simulink model "WT_FFNN_trainbfg_15_15_15_st_5_controller_Oct_6_2023_Nor_0"  (R2021a)
settings: Solver=VariableStepAuto  StartTime=0.0  StopTime=10.0  RelTol=1e-3
libraries: neural x50
(part 2 of 2)

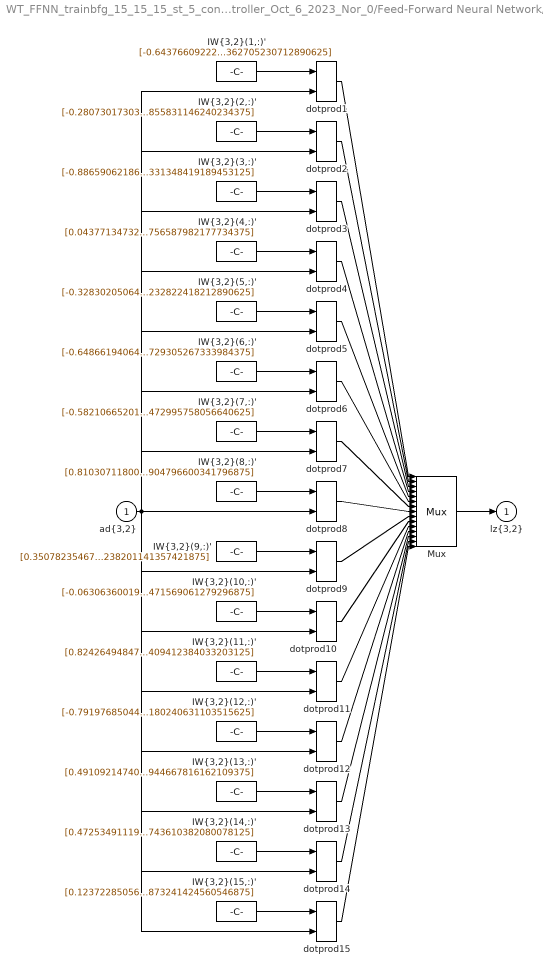
== system WT_FFNN_trainbfg_15_15_15_st_5_controller_Oct_6_2023_Nor_0/Feed-Forward Neural Network/Layer 3/LW{3,2} ==
  "ad{3,2}" : Inport  PortDimensions=15
      mask Display: e = 0.06;c1 = [120 230 180]/255;c2 = ([120 230 180]+0)/(256+128);c3 = ([120 230 180]+128)/(256+128);patch([0 1 1 0],[0 0 1 1],c1);patch([0 1 1 1-e 1-e 0+e],[0 0 1 1-e 0+e 0+e],c2);patch([0 0 1 1-e 0+e 0+e],[0 1 1 1-e 1-e 0+e],c3);plot([0 1 1 0 0],[0 0 1 1 0]);
  "IW{3,2}(1,:)'" : Constant  Value=[-0.643766092226467190329231016221456229686737060546875;-0.63161180496894697711240951321087777614593505859375;-0.0878846663125170124430951545946300029754638671875;0.0675439035340004156893201070488430559635162353515625;0.3850639727730376105085952076478861272335052490234375;-0.897336227775257899708094555535353720188140869140625;0.4800646559755552544856982422061264514923095703125;-0.5886509570704803184781894742627628147602081298828125;-0.7754320756879466980393544872640632092952728271484375;-0.0247924491321527273868241536547429859638214111328125;-0.81529532256159686909313677460886538028717041015625;-0.367142001707418064171406513196416199207305908203125;0.9758694699049907939070180873386561870574951171875;-0.2984465102282147785928145822254009544849395751953125;-0.750254482560374302835271009826101362705230712890625]
      mask Display: e = 0.06;c1 = [120 150 230]/255;c2 = ([120 150 230]+0)/383;c3 = ([120 150 230]+128)/383;patch([0 1 1 0],[0 0 1 1],c1);patch([0 1 1 1-e 1-e 0+e],[0 0 1 1-e 0+e 0+e],c2);patch([0 0 1 1-e 0+e 0+e],[0 1 1 1-e 1-e 0+e],c3);plot([0 1 1 0 0],[0 0 1 1 0]);disp('weights');
  "IW{3,2}(10,:)'" : Constant  Value=[-0.0630636001920052979841102569480426609516143798828125;-0.366578988970010344328187557039200328290462493896484375;0.519459618514004350942059318185783922672271728515625;0.0921458484020575563366861615577363409101963043212890625;-0.7442232404340096696415685073588974773883819580078125;-1.079327489691291219742197426967322826385498046875;0.369217770489993657445637609271216206252574920654296875;-0.601335359818960579758595486055128276348114013671875;0.0032313445087976890197911661317675680038519203662872314453125;-0.896971085063572370899009911227039992809295654296875;-0.6861878613530782988760847729281522333621978759765625;0.68989207606787716908769425572245381772518157958984375;0.07321916960369133364761040638768463395535945892333984375;-0.333963203642246353464173580505303107202053070068359375;0.52767289553089458120638255422818474471569061279296875]
      mask Display: e = 0.06;c1 = [120 150 230]/255;c2 = ([120 150 230]+0)/383;c3 = ([120 150 230]+128)/383;patch([0 1 1 0],[0 0 1 1],c1);patch([0 1 1 1-e 1-e 0+e],[0 0 1 1-e 0+e 0+e],c2);patch([0 0 1 1-e 0+e 0+e],[0 1 1 1-e 1-e 0+e],c3);plot([0 1 1 0 0],[0 0 1 1 0]);disp('weights');
  "IW{3,2}(11,:)'" : Constant  Value=[0.82426494847924569597807931131683290004730224609375;-0.97294544089362500205453443413716740906238555908203125;0.28985203172992990428014081771834753453731536865234375;0.0548147619280814624165287796131451614201068878173828125;0.0990802140303959077982653980143368244171142578125;0.292797576551611538064889828092418611049652099609375;0.58356272391747465722033894053311087191104888916015625;-0.5219904965795241214010502517339773476123809814453125;-0.7694257985340786643035926317679695785045623779296875;-0.3683771233222679075680616733734495937824249267578125;-0.79654204929376859478651340396027080714702606201171875;0.437512109004076332752219968824647367000579833984375;-0.69209100898033104609652355065918527543544769287109375;-0.2746468641281059053227409094688482582569122314453125;0.51865325037653786655056364907068200409412384033203125]
      mask Display: e = 0.06;c1 = [120 150 230]/255;c2 = ([120 150 230]+0)/383;c3 = ([120 150 230]+128)/383;patch([0 1 1 0],[0 0 1 1],c1);patch([0 1 1 1-e 1-e 0+e],[0 0 1 1-e 0+e 0+e],c2);patch([0 0 1 1-e 0+e 0+e],[0 1 1 1-e 1-e 0+e],c3);plot([0 1 1 0 0],[0 0 1 1 0]);disp('weights');
  "IW{3,2}(12,:)'" : Constant  Value=[-0.7919768504412429965810815701843239367008209228515625;1.021337337366363673396563171991147100925445556640625;-1.10070096439400533228081258130259811878204345703125;0.54194625703035803621077093339408747851848602294921875;-0.029541182830081336163630112423561513423919677734375;-0.09421701438622749613660545264792745001614093780517578125;-0.57891826972255999717020813477574847638607025146484375;0.08794848163775025040589383706901571713387966156005859375;1.2460687532080745310025804428732953965663909912109375;0.448536259228720146641222754624322988092899322509765625;-0.88810303508568055885774583657621406018733978271484375;-0.1498027423311489580992628134481492452323436737060546875;0.160199994159698155815618747510598041117191314697265625;-0.257260398151900548935344659184920601546764373779296875;0.48137873566461009122718905928195454180240631103515625]
      mask Display: e = 0.06;c1 = [120 150 230]/255;c2 = ([120 150 230]+0)/383;c3 = ([120 150 230]+128)/383;patch([0 1 1 0],[0 0 1 1],c1);patch([0 1 1 1-e 1-e 0+e],[0 0 1 1-e 0+e 0+e],c2);patch([0 0 1 1-e 0+e 0+e],[0 1 1 1-e 1-e 0+e],c3);plot([0 1 1 0 0],[0 0 1 1 0]);disp('weights');
  "IW{3,2}(13,:)'" : Constant  Value=[0.4910921474034346534409678497468121349811553955078125;-0.48744557436756996704474431680864654481410980224609375;-1.014034144660356684397584103862755000591278076171875;0.4724792507893542659047625420498661696910858154296875;0.7809513583688765248069785229745320975780487060546875;0.5203015162644302193939438438974320888519287109375;-0.6241583092029754364915561382076703011989593505859375;-0.81700253732117555927061403053812682628631591796875;-0.6241863057843290985005069160251878201961517333984375;0.2760602048501932248569801231496967375278472900390625;-0.7697405297430404136349579857778735458850860595703125;-0.45085593242650479073319047529366798698902130126953125;-0.439984497093076132312461368201184086501598358154296875;0.554792900069340788604677072726190090179443359375;0.4873766829746519757549094720161519944667816162109375]
      mask Display: e = 0.06;c1 = [120 150 230]/255;c2 = ([120 150 230]+0)/383;c3 = ([120 150 230]+128)/383;patch([0 1 1 0],[0 0 1 1],c1);patch([0 1 1 1-e 1-e 0+e],[0 0 1 1-e 0+e 0+e],c2);patch([0 0 1 1-e 0+e 0+e],[0 1 1 1-e 1-e 0+e],c3);plot([0 1 1 0 0],[0 0 1 1 0]);disp('weights');
  "IW{3,2}(14,:)'" : Constant  Value=[0.4725349111932770629351807656348682940006256103515625;-0.689178476180853039068097132258117198944091796875;0.2356972366457289747021519588088267482817173004150390625;0.626963724406184308435285856830887496471405029296875;0.597920557625758686270955877262167632579803466796875;0.625541261646222590542265606927685439586639404296875;-1.1026078992220214036734660112415440380573272705078125;-0.19770856332119357556820204990799538791179656982421875;-0.077371211188020871940551614898140542209148406982421875;-0.7870523574073573502829503922839649021625518798828125;-0.669477187150147035055169908446259796619415283203125;-0.9783172116776768234558403491973876953125;0.905331492010126748226639392669312655925750732421875;-0.5450102600935970986739675936405546963214874267578125;-0.7881591665344693797834452198003418743610382080078125]
      mask Display: e = 0.06;c1 = [120 150 230]/255;c2 = ([120 150 230]+0)/383;c3 = ([120 150 230]+128)/383;patch([0 1 1 0],[0 0 1 1],c1);patch([0 1 1 1-e 1-e 0+e],[0 0 1 1-e 0+e 0+e],c2);patch([0 0 1 1-e 0+e 0+e],[0 1 1 1-e 1-e 0+e],c3);plot([0 1 1 0 0],[0 0 1 1 0]);disp('weights');
  "IW{3,2}(15,:)'" : Constant  Value=[0.12372285056327481100879595032893121242523193359375;-0.72140085239758067192639146014698781073093414306640625;0.86439986632040366476559256625478155910968780517578125;-0.59112412850498685656930319964885711669921875;0.4686821673919394637408686321577988564968109130859375;-0.258477290842136608883805592995486222207546234130859375;0.7900688209342423551362344369408674538135528564453125;-1.0831855079199177449567059738910757005214691162109375;0.1882682004181205071002835893523297272622585296630859375;-0.761400721393763912914209868176840245723724365234375;-0.29988241519058600470515330016496591269969940185546875;0.11863292152367811704838373998427414335310459136962890625;0.50817119992942860751128364427131600677967071533203125;-0.366864516161464815358073110473924316465854644775390625;0.362897935872615373664729077063384465873241424560546875]
      mask Display: e = 0.06;c1 = [120 150 230]/255;c2 = ([120 150 230]+0)/383;c3 = ([120 150 230]+128)/383;patch([0 1 1 0],[0 0 1 1],c1);patch([0 1 1 1-e 1-e 0+e],[0 0 1 1-e 0+e 0+e],c2);patch([0 0 1 1-e 0+e 0+e],[0 1 1 1-e 1-e 0+e],c3);plot([0 1 1 0 0],[0 0 1 1 0]);disp('weights');
  "IW{3,2}(2,:)'" : Constant  Value=[-0.2807301730358393587749787911889143288135528564453125;0.19442270067570976976867314078845083713531494140625;-0.7966612127504897333807321047061122953891754150390625;-0.7816915759150828701962154809734784066677093505859375;0.1133396699280251329611246546846814453601837158203125;-0.854229401802047760838831891305744647979736328125;-0.530346170504191416483763532596640288829803466796875;-0.2234567379043965740237354111741296947002410888671875;0.5688557814878254514923128226655535399913787841796875;0.5379165281177382684774102017399854958057403564453125;-0.9843594128613302185470956828794442117214202880859375;-0.564873381154358700229067835607565939426422119140625;-0.6591359538862333611319854753674007952213287353515625;0.3710714174950744403957969552720896899700164794921875;-0.951131967899252028786349910660646855831146240234375]
      mask Display: e = 0.06;c1 = [120 150 230]/255;c2 = ([120 150 230]+0)/383;c3 = ([120 150 230]+128)/383;patch([0 1 1 0],[0 0 1 1],c1);patch([0 1 1 1-e 1-e 0+e],[0 0 1 1-e 0+e 0+e],c2);patch([0 0 1 1-e 0+e 0+e],[0 1 1 1-e 1-e 0+e],c3);plot([0 1 1 0 0],[0 0 1 1 0]);disp('weights');
  "IW{3,2}(3,:)'" : Constant  Value=[-0.8865906218634176383375233854167163372039794921875;-0.4173596361538345345110201378702186048030853271484375;0.94817629014061421965919862486771307885646820068359375;0.382433549701703678902475758150103501975536346435546875;-0.20695841483681487460444259340874850749969482421875;-0.9808227906319275657409662017016671597957611083984375;0.472630354818219744483798194778501056134700775146484375;0.1552047080825973146556151505137677304446697235107421875;-0.5535059857181021669703113730065524578094482421875;-0.26582664726738924887428083820850588381290435791015625;-0.1114708427107084232066114282133639790117740631103515625;-0.5343712969343707985814262428903020918369293212890625;-0.55095411778595515528422765783034265041351318359375;-0.421040236130094502886578311517951078712940216064453125;-0.419775850566837693822463961623725481331348419189453125]
      mask Display: e = 0.06;c1 = [120 150 230]/255;c2 = ([120 150 230]+0)/383;c3 = ([120 150 230]+128)/383;patch([0 1 1 0],[0 0 1 1],c1);patch([0 1 1 1-e 1-e 0+e],[0 0 1 1-e 0+e 0+e],c2);patch([0 0 1 1-e 0+e 0+e],[0 1 1 1-e 1-e 0+e],c3);plot([0 1 1 0 0],[0 0 1 1 0]);disp('weights');
  "IW{3,2}(4,:)'" : Constant  Value=[0.0437713473225584959180878286133520305156707763671875;-0.7804216873352183281298266592784784734249114990234375;-0.2787118030579514016409348187153227627277374267578125;-0.201163548237447697974999982761801220476627349853515625;-0.8768186658920706921804821831756271421909332275390625;0.69390680565058027173819255040143616497516632080078125;0.97507725501613740082262893338338471949100494384765625;-0.55942047888349455408985022586421109735965728759765625;0.278239923091626539797260875275242142379283905029296875;-0.450913782201801727200773939330247230827808380126953125;0.411797200423771936339534249782445840537548065185546875;0.836294422102941581442792084999382495880126953125;-0.216248531117989362115849871770478785037994384765625;0.1093947460428724427483615500023006461560726165771484375;-0.365005400146794778404313319697394035756587982177734375]
      mask Display: e = 0.06;c1 = [120 150 230]/255;c2 = ([120 150 230]+0)/383;c3 = ([120 150 230]+128)/383;patch([0 1 1 0],[0 0 1 1],c1);patch([0 1 1 1-e 1-e 0+e],[0 0 1 1-e 0+e 0+e],c2);patch([0 0 1 1-e 0+e 0+e],[0 1 1 1-e 1-e 0+e],c3);plot([0 1 1 0 0],[0 0 1 1 0]);disp('weights');
  "IW{3,2}(5,:)'" : Constant  Value=[-0.3283020506461509224749306667945347726345062255859375;-1.0756667734631670807488035279675386846065521240234375;-0.44430709094670317593767094876966439187526702880859375;-0.6985551875055742154785320963128469884395599365234375;0.5603510629823471589361361111514270305633544921875;0.5762260002307371120622292437474243342876434326171875;0.8291722243223598187711331775062717497348785400390625;0.1374628424309248531098859302801429294049739837646484375;0.74139743393488355405196443825843743979930877685546875;-0.92553073185934398026120106806047260761260986328125;0.68564812657096230186226648584124632179737091064453125;0.2073458705438895599559856464111362583935260772705078125;-1.2029327427730522881432762005715630948543548583984375;0.7879912065605456650274618368712253868579864501953125;0.307245991826452069517472409643232822418212890625]
      mask Display: e = 0.06;c1 = [120 150 230]/255;c2 = ([120 150 230]+0)/383;c3 = ([120 150 230]+128)/383;patch([0 1 1 0],[0 0 1 1],c1);patch([0 1 1 1-e 1-e 0+e],[0 0 1 1-e 0+e 0+e],c2);patch([0 0 1 1-e 0+e 0+e],[0 1 1 1-e 1-e 0+e],c3);plot([0 1 1 0 0],[0 0 1 1 0]);disp('weights');
  "IW{3,2}(6,:)'" : Constant  Value=[-0.6486619406486784367160680631059221923351287841796875;0.78230111669044222200142257861443795263767242431640625;-0.89586528370598073056640942013473249971866607666015625;0.27952203311936407725823983128066174685955047607421875;-0.3248322718959097965552018649759702384471893310546875;0.11315719229489339114902435312615125440061092376708984375;-0.82755402606266958986935833308962173759937286376953125;-0.03089175723395513883939855759308557026088237762451171875;-0.362530144589864544713009308907203376293182373046875;0.35108497343814704105824375801603309810161590576171875;-0.161769639677050214299214303537155501544475555419921875;0.04734728740250859768678992622881196439266204833984375;0.479859734087550615644346407862030901014804840087890625;0.047514877164076228799327594742862856946885585784912109375;0.91387184814136812605056547909043729305267333984375]
      mask Display: e = 0.06;c1 = [120 150 230]/255;c2 = ([120 150 230]+0)/383;c3 = ([120 150 230]+128)/383;patch([0 1 1 0],[0 0 1 1],c1);patch([0 1 1 1-e 1-e 0+e],[0 0 1 1-e 0+e 0+e],c2);patch([0 0 1 1-e 0+e 0+e],[0 1 1 1-e 1-e 0+e],c3);plot([0 1 1 0 0],[0 0 1 1 0]);disp('weights');
  "IW{3,2}(7,:)'" : Constant  Value=[-0.582106652013729242156614418490789830684661865234375;-0.8570943744259109653427231023670174181461334228515625;-0.40351205622447228194005219847895205020904541015625;-0.979326763313207226957501916331239044666290283203125;0.215731814525891518741218533250503242015838623046875;-0.735834088572874467359952177503146231174468994140625;-0.2671267673616022353400012434576638042926788330078125;-0.6963089497674668226778749158256687223911285400390625;0.3895043892358802661846084447461180388927459716796875;-0.14087108149629390396739836432971060276031494140625;-0.782364123453909154903840317274443805217742919921875;-0.631132664484693517437108312151394784450531005859375;-0.19522333460767615775921512977220118045806884765625;-0.3293773385895077954188536750734783709049224853515625;0.8714617455697608594533676296123303472995758056640625]
      mask Display: e = 0.06;c1 = [120 150 230]/255;c2 = ([120 150 230]+0)/383;c3 = ([120 150 230]+128)/383;patch([0 1 1 0],[0 0 1 1],c1);patch([0 1 1 1-e 1-e 0+e],[0 0 1 1-e 0+e 0+e],c2);patch([0 0 1 1-e 0+e 0+e],[0 1 1 1-e 1-e 0+e],c3);plot([0 1 1 0 0],[0 0 1 1 0]);disp('weights');
  "IW{3,2}(8,:)'" : Constant  Value=[0.8103071180089280733938039702479727566242218017578125;-0.7595903776732757517464733609813265502452850341796875;-1.031993112604987938851763829006813466548919677734375;-0.9607340944964324336297067929990589618682861328125;0.4825080990044359197099765879102051258087158203125;0.649925746808536874965511742630042135715484619140625;-0.218869966380718927734250200956012122333049774169921875;0.56386445722714151340682064983411692082881927490234375;0.6203199928330802581655234462232328951358795166015625;-0.09692252373331723680482951976955519057810306549072265625;0.278899550446603139430834517042967490851879119873046875;-0.65482024986183262615924149940838105976581573486328125;0.7599689320797693437015141171286813914775848388671875;-0.15051776628284063708207440868136473000049591064453125;-0.084227332291266332475743183749727904796600341796875]
      mask Display: e = 0.06;c1 = [120 150 230]/255;c2 = ([120 150 230]+0)/383;c3 = ([120 150 230]+128)/383;patch([0 1 1 0],[0 0 1 1],c1);patch([0 1 1 1-e 1-e 0+e],[0 0 1 1-e 0+e 0+e],c2);patch([0 0 1 1-e 0+e 0+e],[0 1 1 1-e 1-e 0+e],c3);plot([0 1 1 0 0],[0 0 1 1 0]);disp('weights');
  "IW{3,2}(9,:)'" : Constant  Value=[0.35078235467249374579523646389134228229522705078125;-0.892491215582572383624437861726619303226470947265625;0.010856284915405911561947505106218159198760986328125;0.3358322431472473557079183592577464878559112548828125;-0.7903735160530007686219278184580616652965545654296875;-0.7792930387153027549373973670299164950847625732421875;0.3700569453232185335167514494969509541988372802734375;-0.7987873552751569850016721829888410866260528564453125;-0.1347153477057989601206600127625279128551483154296875;0.2197143385804321003007544277352280914783477783203125;-0.7470002693413941852185189418378286063671112060546875;-0.8453063837746463971001276149763725697994232177734375;-0.195632029555030673151350129046477377414703369140625;-0.0948149168613519055526239753817208111286163330078125;-0.5190432063358307868128349582548253238201141357421875]
      mask Display: e = 0.06;c1 = [120 150 230]/255;c2 = ([120 150 230]+0)/383;c3 = ([120 150 230]+128)/383;patch([0 1 1 0],[0 0 1 1],c1);patch([0 1 1 1-e 1-e 0+e],[0 0 1 1-e 0+e 0+e],c2);patch([0 0 1 1-e 0+e 0+e],[0 1 1 1-e 1-e 0+e],c3);plot([0 1 1 0 0],[0 0 1 1 0]);disp('weights');
  Mux : Mux  Inputs=15
      mask Display: e = 0.06;c1 = [120 150 230]/255;c2 = ([120 150 230]+0)/383;c3 = ([120 150 230]+128)/383;patch([0 1 1 0],[0 0 1 1],c1);patch([0 1 1 1-e 1-e 0+e],[0 0 1 1-e 0+e 0+e],c2);patch([0 0 1 1-e 0+e 0+e],[0 1 1 1-e 1-e 0+e],c3);plot([0 1 1 0 0],[0 0 1 1 0]);disp('Mux');
  dotprod{1..15} (15 alike) : neural/Weight Functions/dotprod
  "lz{3,2}" : Outport
      mask Display: e = 0.06;c1 = [120 230 180]/255;c2 = ([120 230 180]+0)/(256+128);c3 = ([120 230 180]+128)/(256+128);patch([0 1 1 0],[0 0 1 1],c1);patch([0 1 1 1-e 1-e 0+e],[0 0 1 1-e 0+e 0+e],c2);patch([0 0 1 1-e 0+e 0+e],[0 1 1 1-e 1-e 0+e],c3);plot([0 1 1 0 0],[0 0 1 1 0]);
  wires:
  "IW{3,2}(1,:)'"/1 -> dotprod1/1
  "ad{3,2}"/1 -> dotprod1/2, dotprod2/2, dotprod3/2, dotprod4/2, dotprod5/2, dotprod6/2, dotprod7/2, dotprod8/2, dotprod9/2, dotprod10/2, dotprod11/2, dotprod12/2, dotprod13/2, dotprod14/2, dotprod15/2
  dotprod1/1 -> Mux/1
  "IW{3,2}(2,:)'"/1 -> dotprod2/1
  dotprod2/1 -> Mux/2
  "IW{3,2}(3,:)'"/1 -> dotprod3/1
  dotprod3/1 -> Mux/3
  "IW{3,2}(4,:)'"/1 -> dotprod4/1
  dotprod4/1 -> Mux/4
  "IW{3,2}(5,:)'"/1 -> dotprod5/1
  dotprod5/1 -> Mux/5
  "IW{3,2}(6,:)'"/1 -> dotprod6/1
  dotprod6/1 -> Mux/6
  "IW{3,2}(7,:)'"/1 -> dotprod7/1
  dotprod7/1 -> Mux/7
  "IW{3,2}(8,:)'"/1 -> dotprod8/1
  dotprod8/1 -> Mux/8
  "IW{3,2}(9,:)'"/1 -> dotprod9/1
  dotprod9/1 -> Mux/9
  "IW{3,2}(10,:)'"/1 -> dotprod10/1
  dotprod10/1 -> Mux/10
  "IW{3,2}(11,:)'"/1 -> dotprod11/1
  dotprod11/1 -> Mux/11
  "IW{3,2}(12,:)'"/1 -> dotprod12/1
  dotprod12/1 -> Mux/12
  "IW{3,2}(13,:)'"/1 -> dotprod13/1
  dotprod13/1 -> Mux/13
  "IW{3,2}(14,:)'"/1 -> dotprod14/1
  dotprod14/1 -> Mux/14
  "IW{3,2}(15,:)'"/1 -> dotprod15/1
  dotprod15/1 -> Mux/15
  Mux/1 -> "lz{3,2}"/1

== system WT_FFNN_trainbfg_15_15_15_st_5_controller_Oct_6_2023_Nor_0/Feed-Forward Neural Network/Layer 4/Delays 1 ==
  "p{4}" : Inport  PortDimensions=15
      mask Display: e = 0.06;c1 = [120 230 180]/255;c2 = ([120 230 180]+0)/(256+128);c3 = ([120 230 180]+128)/(256+128);patch([0 1 1 0],[0 0 1 1],c1);patch([0 1 1 1-e 1-e 0+e],[0 0 1 1-e 0+e 0+e],c2);patch([0 0 1 1-e 0+e 0+e],[0 1 1 1-e 1-e 0+e],c3);plot([0 1 1 0 0],[0 0 1 1 0]);
  mux : Mux  Inputs=1
      mask Display: e = 0.06;c1 = [120 150 230]/255;c2 = ([120 150 230]+0)/383;c3 = ([120 150 230]+128)/383;patch([0 1 1 0],[0 0 1 1],c1);patch([0 1 1 1-e 1-e 0+e],[0 0 1 1-e 0+e 0+e],c2);patch([0 0 1 1-e 0+e 0+e],[0 1 1 1-e 1-e 0+e],c3);plot([0 1 1 0 0],[0 0 1 1 0]);disp('Mux')
  "pd{4,3}" : Outport
      mask Display: e = 0.06;c1 = [120 230 180]/255;c2 = ([120 230 180]+0)/(256+128);c3 = ([120 230 180]+128)/(256+128);patch([0 1 1 0],[0 0 1 1],c1);patch([0 1 1 1-e 1-e 0+e],[0 0 1 1-e 0+e 0+e],c2);patch([0 0 1 1-e 0+e 0+e],[0 1 1 1-e 1-e 0+e],c3);plot([0 1 1 0 0],[0 0 1 1 0]);
  wires:
  "p{4}"/1 -> mux/1
  mux/1 -> "pd{4,3}"/1

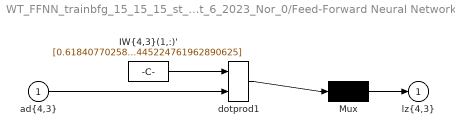
== system WT_FFNN_trainbfg_15_15_15_st_5_controller_Oct_6_2023_Nor_0/Feed-Forward Neural Network/Layer 4/LW{4,3} ==
  "ad{4,3}" : Inport  PortDimensions=15
      mask Display: e = 0.06;c1 = [120 230 180]/255;c2 = ([120 230 180]+0)/(256+128);c3 = ([120 230 180]+128)/(256+128);patch([0 1 1 0],[0 0 1 1],c1);patch([0 1 1 1-e 1-e 0+e],[0 0 1 1-e 0+e 0+e],c2);patch([0 0 1 1-e 0+e 0+e],[0 1 1 1-e 1-e 0+e],c3);plot([0 1 1 0 0],[0 0 1 1 0]);
  "IW{4,3}(1,:)'" : Constant  Value=[0.61840770258758670507859278586693108081817626953125;0.4972377435523942512674011595663614571094512939453125;-0.73197087610976818705665891684475354850292205810546875;-0.284320000349995549715487186404061503708362579345703125;-0.55021885195268549484381992442649789154529571533203125;0.454230957654833955583484339513233862817287445068359375;-0.20223849523360204472055556834675371646881103515625;-1.091113431875989636665735815768130123615264892578125;-0.63852447949041124530822344240732491016387939453125;-0.50407679792810144991932475022622384130954742431640625;-0.96433255355675273623461407623835839331150054931640625;1.6878212913382439896992082140059210360050201416015625;0.70060147910711922936144446794060058891773223876953125;1.2562341623264738910137339189532212913036346435546875;-0.97480569835202468542689757668995298445224761962890625]
      mask Display: e = 0.06;c1 = [120 150 230]/255;c2 = ([120 150 230]+0)/383;c3 = ([120 150 230]+128)/383;patch([0 1 1 0],[0 0 1 1],c1);patch([0 1 1 1-e 1-e 0+e],[0 0 1 1-e 0+e 0+e],c2);patch([0 0 1 1-e 0+e 0+e],[0 1 1 1-e 1-e 0+e],c3);plot([0 1 1 0 0],[0 0 1 1 0]);disp('weights');
  Mux : Mux  Inputs=1
      mask Display: e = 0.06;c1 = [120 150 230]/255;c2 = ([120 150 230]+0)/383;c3 = ([120 150 230]+128)/383;patch([0 1 1 0],[0 0 1 1],c1);patch([0 1 1 1-e 1-e 0+e],[0 0 1 1-e 0+e 0+e],c2);patch([0 0 1 1-e 0+e 0+e],[0 1 1 1-e 1-e 0+e],c3);plot([0 1 1 0 0],[0 0 1 1 0]);disp('Mux');
  dotprod1 : neural/Weight Functions/dotprod
  "lz{4,3}" : Outport
      mask Display: e = 0.06;c1 = [120 230 180]/255;c2 = ([120 230 180]+0)/(256+128);c3 = ([120 230 180]+128)/(256+128);patch([0 1 1 0],[0 0 1 1],c1);patch([0 1 1 1-e 1-e 0+e],[0 0 1 1-e 0+e 0+e],c2);patch([0 0 1 1-e 0+e 0+e],[0 1 1 1-e 1-e 0+e],c3);plot([0 1 1 0 0],[0 0 1 1 0]);
  wires:
  "IW{4,3}(1,:)'"/1 -> dotprod1/1
  "ad{4,3}"/1 -> dotprod1/2
  dotprod1/1 -> Mux/1
  Mux/1 -> "lz{4,3}"/1
